simulink model "RR_instability"  (R2020b)
settings: Solver=FixedStepAuto  StartTime=0  StopTime=10.0  FixedStep=0.001  MaxStep=0.05  RelTol=1e-3
values from neighbouring files (symbols this model uses):
  e_max = 0.01    [init.m]
  F_int_max = [5;5]    [init.m]
  F_max = [1;1]    [init.m]
  g = 9.81    [init.m]
  I1 = evalin('base','I1')    [Mass.m]    (also in init.m = 1)
  I2 = evalin('base','I2')    [Mass.m]    (also in init.m = 1)
  l1 = evalin('base','l1')    [Mass.m]    (also in init.m = 1)
  l2 = evalin('base','l2')    [Mass.m]    (also in init.m = 1)
  m1 = evalin('base','m1')    [Mass.m]    (also in init.m = 1)
  m2 = evalin('base','m2')    [Mass.m]    (also in init.m = 1)
  mass = 1    [init.m]
  ts_bound = 0.05    [init.m]
libraries: cstblocks x2, simulink x1
settings Model: Creator=chiara-s  LastModifiedBy=chiara-s

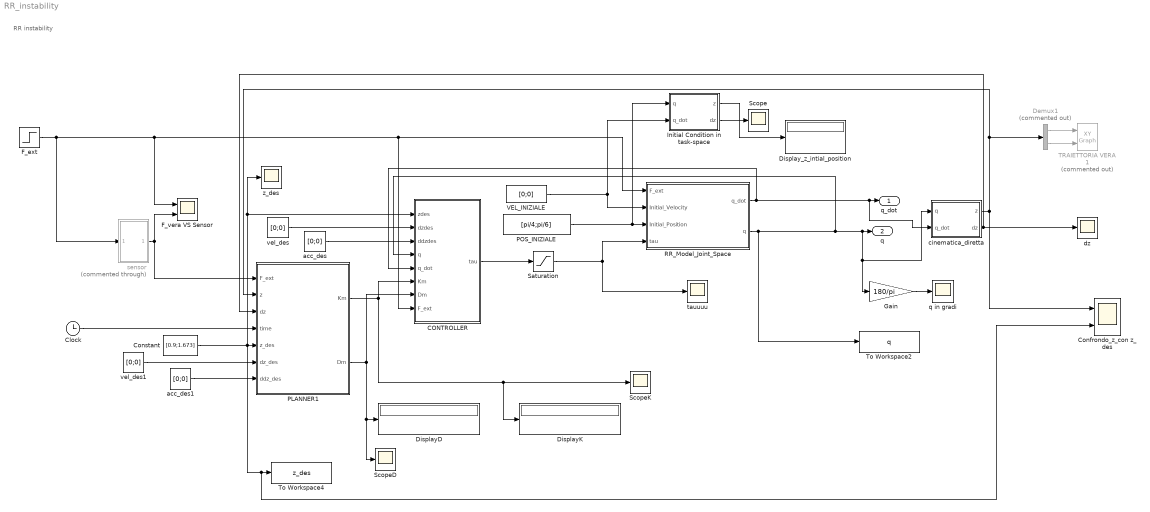
== system RR_instability ==
  note: RR instability
  CONTROLLER : MATLAB Function  TreatAsAtomicUnit=on
  Clock : Clock
  Confrondo_z_con z_des : Scope  NumInputPorts=2
  Constant : Constant  Value=[0.9;1.673]
  Demux1 : Demux  Commented=on  Outputs=2
  DisplayD : Display
  DisplayK : Display
  Display_z_intial_position : Display
  F_ext : Step  Before=[0;0]  After=[0;0]  SampleTime=0
  F_vera VS Sensor : Scope  NumInputPorts=2
  Gain : Gain  Gain=180/pi
  Initial Condition in task-space : MATLAB Function  TreatAsAtomicUnit=on
  PLANNER1 : MATLAB Function  TreatAsAtomicUnit=on
  POS_INIZIALE : Constant  Value=[pi/4;pi/6]
  RR_Model_Joint_Space : Subsystem
  Saturation : Saturate  UpperLimit=1000  LowerLimit=-1000
  Scope : Scope
  ScopeD : Scope
  ScopeK : Scope
  TRAIETTORIA VERA 1 : simulink/Sinks/XY Graph  Commented=on  xmin=-2  xmax=2  ymin=-2  ymax=2  st=-1
  To Workspace2 : ToWorkspace  VariableName=q  SaveFormat=Structure With Time  SampleTime=-1
      settings: Save2DSignal=2-D array (concatenate along first dimension)
  To Workspace4 : ToWorkspace  VariableName=z_des  SaveFormat=Structure With Time  SampleTime=0.001
      settings: Save2DSignal=2-D array (concatenate along first dimension)
  VEL_INIZIALE : Constant  Value=[0;0]
  acc_des : Constant  Value=[0;0]
  acc_des1 : Constant  Value=[0;0]
  cinematica_diretta : MATLAB Function  TreatAsAtomicUnit=on
  dz : Scope
  q in gradi : Scope
  sensor : Subsystem  Commented=through
  tauuuu : Scope
  vel_des : Constant  Value=[0;0]
  vel_des1 : Constant  Value=[0;0]
  z_des : Scope
  q_dot : Outport
  q : Outport  Port=2
  wires:
  RR_Model_Joint_Space/1(q_dot) -> cinematica_diretta/2(q_dot), q_dot/1, CONTROLLER/5(q_dot)
  Initial Condition in task-space/1(z) -> Display_z_intial_position/1
  F_ext/1 -> sensor/1(In1), RR_Model_Joint_Space/1(F_ext), CONTROLLER/8(F_ext), F_vera VS Sensor/1
  PLANNER1/1(Km) -> ScopeK/1, DisplayK/1, CONTROLLER/6(Km)
  vel_des/1 -> CONTROLLER/2(dzdes)
  Demux1/2 -> TRAIETTORIA VERA 1/2
  PLANNER1/2(Dm) -> CONTROLLER/7(Dm), ScopeD/1, DisplayD/1
  RR_Model_Joint_Space/2(q) -> CONTROLLER/4(q), Gain/1, cinematica_diretta/1(q), q/1, To Workspace2/1
  Demux1/1 -> TRAIETTORIA VERA 1/1
  cinematica_diretta/1(z) -> PLANNER1/2(z), Demux1/1, Confrondo_z_con z_des/1
  cinematica_diretta/2(dz) -> PLANNER1/3(dz), dz/1
  POS_INIZIALE/1 -> RR_Model_Joint_Space/3(Initial_Position), Initial Condition in task-space/1(q)
  Gain/1 -> q in gradi/1
  VEL_INIZIALE/1 -> Initial Condition in task-space/2(q_dot), RR_Model_Joint_Space/2(Initial_Velocity)
  acc_des/1 -> CONTROLLER/3(ddzdes)
  Initial Condition in task-space/2(dz) -> Scope/1
  Clock/1 -> PLANNER1/4(time)
  sensor/1(Out1) -> PLANNER1/1(F_ext), F_vera VS Sensor/2
  Constant/1 -> Confrondo_z_con z_des/2, To Workspace4/1, z_des/1, CONTROLLER/1(zdes), PLANNER1/5(z_des)
  vel_des1/1 -> PLANNER1/6(dz_des)
  acc_des1/1 -> PLANNER1/7(ddz_des)
  CONTROLLER/1(tau) -> Saturation/1
  Saturation/1 -> RR_Model_Joint_Space/4(tau), tauuuu/1

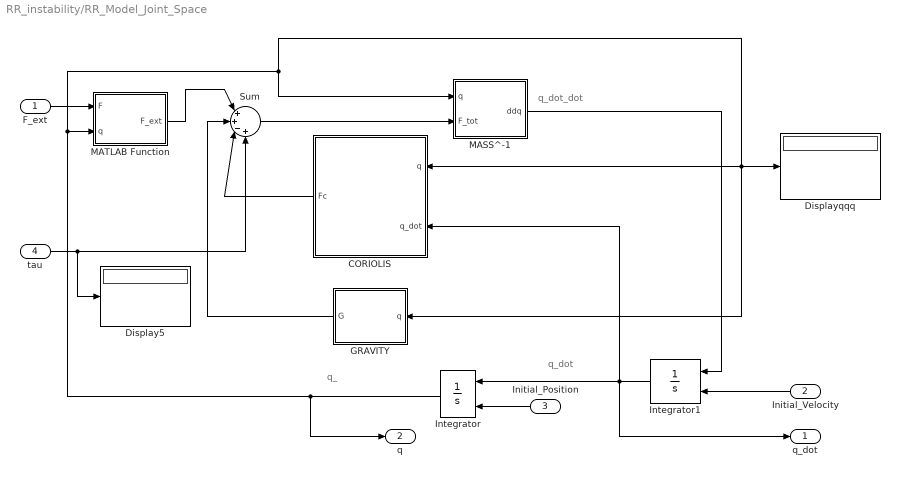
== system RR_instability/RR_Model_Joint_Space ==
  note: q_dot
  note: q_dot_dot
  note: q_
  F_ext : Inport
  Initial_Velocity : Inport  Port=2
  Initial_Position : Inport  Port=3
  tau : Inport  Port=4
  CORIOLIS : MATLAB Function  TreatAsAtomicUnit=on
  Display5 : Display
  Displayqqq : Display
  GRAVITY : MATLAB Function  TreatAsAtomicUnit=on
  Integrator : Integrator  InitialConditionSource=external
  Integrator1 : Integrator  InitialConditionSource=external  InitialCondition=[0;0]
  MASS^-1 : MATLAB Function  TreatAsAtomicUnit=on
  MATLAB Function : MATLAB Function  TreatAsAtomicUnit=on
  Sum : Sum  Inputs=|++-+
  q_dot : Outport
  q : Outport  Port=2
  wires:
  GRAVITY/1(G) -> Sum/2
  MATLAB Function/1(F_ext) -> Sum/1
  Initial_Position/1 -> Integrator/2
  F_ext/1 -> MATLAB Function/1(F)
  Integrator/1 -> MASS^-1/1(q), GRAVITY/1(q), Displayqqq/1, CORIOLIS/1(q), MATLAB Function/2(q), q/1
  Integrator1/1 -> q_dot/1, CORIOLIS/2(q_dot), Integrator/1
  Initial_Velocity/1 -> Integrator1/2
  MASS^-1/1(ddq) -> Integrator1/1
  Sum/1 -> MASS^-1/2(F_tot)
  CORIOLIS/1(Fc) -> Sum/3
  tau/1 -> Display5/1, Sum/4

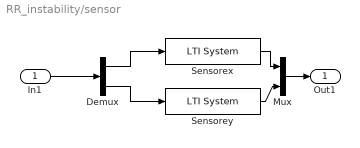
== system RR_instability/sensor ==
  In1 : Inport
  Demux : Demux  Outputs=2
  Mux : Mux  Inputs=2
  Sensorex : cstblocks/LTI System  sys=tf(50^2,[1 0.3*2*50 50^2])  IC=[]
  Sensorey : cstblocks/LTI System  sys=tf(50^2,[1 0.3*2*50 50^2])  IC=[]
  Out1 : Outport
  wires:
  Demux/1 -> Sensorex/1
  Sensorex/1 -> Mux/1
  Sensorey/1 -> Mux/2
  Mux/1 -> Out1/1
  Demux/2 -> Sensorey/1
  In1/1 -> Demux/1

== matlab function RR_instability/RR_Model_Joint_Space/MATLAB Function ==
  data: F input size=2; F_ext output double size=2; q input size=2; l1 parameter; l2 parameter
function F_ext = fcn(F,q,l1, l2)


Ja = [-l1*sin(q(1)) - l2*sin(q(1)+q(2)), -l2*sin(q(1)+q(2)); ...
    l1*cos(q(1)) + l2*cos(q(1)+q(2)), l2*cos(q(1)+q(2))];

F_ext = Ja'*F;

end

== matlab function RR_instability/cinematica_diretta ==
  data: q input double size=2; q_dot input double size=2; z output double size=2; dz output double size=2; l1 parameter; l2 parameter
function [z,dz] = fcn(q,q_dot,l1, l2)

z = zeros(2,1);
z(1) = l1*cos(q(1)) + l2*cos(q(1)+q(2));
z(2) = l1*sin(q(1)) + l2*sin(q(1)+q(2));

Ja = zeros(2,2);
Ja = [-l1*sin(q(1)) - l2*sin(q(1)+q(2)), -l2*sin(q(1)+q(2)); ...
    l1*cos(q(1)) + l2*cos(q(1)+q(2)), l2*cos(q(1)+q(2))];

dz = zeros(2,1);
dz = Ja*q_dot;

end

== matlab function RR_instability/PLANNER1 ==
  settings: updateMethod=DISCRETE
  data: F_max parameter; Km output; Dm output; e_max parameter; F_ext input; z input; dz input; time input; z_des input; dz_des input; ddz_des input; F_int_max parameter; mass parameter; ts_bound parameter
function [Km,Dm] = fcn(F_max, e_max,F_ext, z, dz, time, z_des, dz_des, ddz_des, F_int_max, mass, ts_bound)

%% Description
% decrease k after contact is sensed to limit the interaction force

%% Outputs
% Km            stiffness matrix
% Dm            damping matrix

%% Inputs
% time          current simulation time
% F_ext         measured external force
% mass          mass scalar value 
% F_int_max     desired interaction force
% z_des, dz_des, ddz_des                    desired trajectory
% z             current position
% F_max         estimated force disturbances
% e_max         maximum steady-state error

persistent F_prec kx0 ky0 dx dy t_changex t_changey t_settlx t_settly t_interaction

% time of a first interaction
if isempty(t_interaction)
    t_interaction = 1000;
end

% settling time
if isempty(t_settlx)
    t_settlx = 0;
end
if isempty(t_settly)
    t_settly = 0;
end

% time of last stiffness update
if isempty(t_changex)
    t_changex = 1000;
end
if isempty(t_changey)
    t_changey = 1000;
end

% previous measured force
if isempty(F_prec)
    F_prec = [0;0];
end

% initialization of k and d 
if isempty(kx0)
   kx0 = F_max(1)/e_max; 
end
if isempty(ky0)
   ky0 = F_max(2)/e_max;
end
if isempty(dx)
    dx = sqrt(4*kx0*mass)/10;
end
if isempty(dy)
    dy = sqrt(4*ky0*mass)/10;
end

kx = kx0 - (kx0/2)*sign(dz(1)*(z(1)-z_des(1)));                      %instability
ky = ky0 - (ky0/2)*sign(dz(2)*(z(2)-z_des(2)));

Dm = diag([dx,dy]);
Km = diag([kx,ky]);
end


% kx = kx0;
% ky = ky0;


% if abs(z(1)) < 0.001
%     if t_interaction == 1000
%         t_interaction = time;
%     end
% end
% if time >= t_interaction
%% k continuo
%     t = kx0/2;
%     kx = kx0 + t*(dz(1))*(z(1)-z_des(1));         %    antibouncing x !!!! K bello 
%     ky = ky0 + t*(dz(2))*(z(2)-z_des(2));         %    antibouncing y !!!!

%% instability

%% k discreto
%        kx = kx0 + (kx0/2)*sign(dz(1)*(z(1)-z_des(1)));                    % antibouncing --> K BRUTTO
%        ky = ky0 + (ky0/2)*sign(dz(2)*(z(2)-z_des(2)));

% end




% set final values

== matlab function RR_instability/CONTROLLER ==
  data: zdes input size=2; tau output double size=2; dzdes input size=2; ddzdes input size=2; q input size=2; q_dot input size=2; Km input; Dm input; F_ext input; M parameter
function tau = fcn(zdes, dzdes, ddzdes, q, q_dot, Km, Dm, F_ext, M)
%% PROBLEMA MATRICE DELLE MASSE NON DIAGONALE
coder.extrinsic('Jacobianoa','Jacobianoa_dot','Mass','Coriolis','Gravity','cin_dir')
dz = zeros(2,1);
z = zeros(2,1);
B = zeros(2,2);
S = zeros(2,2);
G = zeros(2,1);
Ja = zeros(2,2);
Ja_dot = zeros(2,2);
Bm = [M 0; 0 M];
Ja = Jacobianoa(q);
Ja_dot = Jacobianoa_dot(q,q_dot);

dz = Ja*q_dot;
z = cin_dir(q);

t = 0.1;
if (deg2rad(-0.1) < q(2)) && (q(2) < deg2rad(0.1)) || (deg2rad(179.9) < q(2)) && (q(2) < deg2rad(180.1)) || (deg2rad(-180.1) < q(2)) && (q(2) < deg2rad(-179.9))
    Ja_inv = (Ja')*inv(Ja*(Ja') + t^2*eye(2,2)); % Damp least square Jacobian method
else 
    Ja_inv = inv(Ja);
end

% Ja_inv = inv(Ja);

B = Mass(q);
Bx = (Ja_inv')* B * Ja_inv;
S = Coriolis(q,q_dot);
G = Gravity(q);
I = eye(2,2);
% tau = B * Ja_inv*(ddzdes - Ja_dot*q_dot) + ...
%     S*q_dot + (Ja')*(Dm*(dzdes - dz) + Km*(zdes- z)) + G;

tau = B*Ja_inv*(ddzdes - Ja_dot*q_dot + ...
    inv(Bm)*(Dm*(dzdes - dz) + Km*(zdes- z))) + S*q_dot - G + ...
    (Ja')*(Bx*inv(Bm) - I)*F_ext;

end

== matlab function RR_instability/Initial Condition in task-space ==
  data: q input double size=2; q_dot input double size=2; z output double size=2; dz output double size=2; l1 parameter; l2 parameter
function [z,dz] = fcn(q,q_dot,l1, l2)

z = zeros(2,1);
z(1) = l1*cos(q(1)) + l2*cos(q(1)+q(2));
z(2) = l1*sin(q(1)) + l2*sin(q(1)+q(2));

Ja = zeros(2,2);
Ja = [-l1*sin(q(1)) - l2*sin(q(1)+q(2)), -l2*sin(q(1)+q(2)); ...
    l1*cos(q(1)) + l2*cos(q(1)+q(2)), l2*cos(q(1)+q(2))];

dz = zeros(2,1);
dz = Ja*q_dot;

end

== matlab function RR_instability/RR_Model_Joint_Space/CORIOLIS ==
  data: q input size=2; Fc output double size=2; q_dot input size=2; a parameter
function Fc = fcn(q,q_dot,a)

C = zeros(2,2);
C = [-a*sin(q(2))*q_dot(2), -a*sin(q(2))*q_dot(1)-a*sin(q(2)*q_dot(2)); ...
    a*sin(q(2))*q_dot(1), 0];

Fc = C*q_dot;

end

== matlab function RR_instability/RR_Model_Joint_Space/GRAVITY ==
  data: q input size=2; G output double size=2; g parameter; l1 parameter; l2 parameter; m1 parameter; m2 parameter
function G = fcn(q,g, l1, l2, m1, m2)


G = [-(l1/2)*cos(q(1))*m1*g - m2*g*(l1*cos(q(1))+(l2/2)*cos(q(1)+q(2))); ...
    -m2*g*(l2/2)*cos(q(1)+q(2))];

end

== matlab function RR_instability/RR_Model_Joint_Space/MASS^-1 ==
  data: q input size=2; ddq output size=2; F_tot input double size=2; I1 parameter; I2 parameter; l1 parameter; l2 parameter; m1 parameter; m2 parameter
function ddq = fcn(q,F_tot,I1, I2, l1, l2, m1, m2)


B = [((l1^2)/4)*m1 + I1 + m2*(l1^2) + m2*((l2^2)/4) + m2*l1*l2*cos(q(2)) + I2, m2*(((l1*l2)/2)*cos(q(2)) + (l2^2)/4) + I2; ...
    m2*(((l1*l2)/2)*cos(q(2)) + (l2^2)/4) + I2, m2*(l2^2)/4 + I2];


ddq = B\F_tot;                      % Ftot*M^-1

end
